simulink model "SVC"  (R2020a)
settings: Solver=VariableStepAuto  StartTime=0.0  StopTime=1  RelTol=1e-3
libraries: powerlib x7, powerlib_meascontrol x2, factslib x1
settings Model: Creator=Naeem Mohammad  LastModifiedBy=Naeem Mohammad

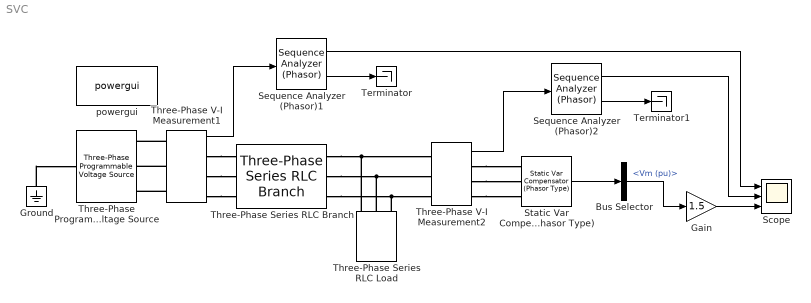
== system SVC ==
  Bus Selector : BusSelector  OutputSignals=Control.Vm (pu)
  Gain : Gain  Gain=1.5
  Ground : powerlib/Elements/Ground  LConnTagsString=a
      settings: SourceProductBaseCode=MT,PS
  Scope : Scope  NumInputPorts=3
  Sequence Analyzer (Phasor)1 : powerlib_meascontrol/Measurements/Sequence Analyzer (Phasor)  seq=Positive
      settings: SourceProductBaseCode=MT,PS
  Sequence Analyzer (Phasor)2 : powerlib_meascontrol/Measurements/Sequence Analyzer (Phasor)  seq=Positive
      settings: SourceProductBaseCode=MT,PS
  Static Var Compensator (Phasor Type) : factslib/Power-Electronics Based FACTS/Static Var Compensator (Phasor Type)  Seq1_Only=on  SystemNominal="[220  60]"  Pbase=200  Qnom="[200  -200]"  Td=4e-3  mode=Voltage regulation  Vref=1  ExternalVref=off  Xs=0.03  Kp_Ki=[0 300]  Bref=0.0
      settings: SourceProductBaseCode=PS
  Terminator : Terminator
  Terminator1 : Terminator
  Three-Phase Series RLC Branch : powerlib/Elements/Three-Phase Series RLC Branch  LConnTagsString=A|B|C  RConnTagsString=A|B|C  BranchType=RC  Resistance=220^2/300  Inductance=220^2/300/(2*pi*60)  Capacitance=(220^2/300)*(2*pi*60)  Measurements=None
      settings: SourceProductBaseCode=MT,PS
  Three-Phase Series RLC Load : powerlib/Elements/Three-Phase Series RLC Load  LConnTagsString=A|B|C  Configuration=Y (grounded)  NominalVoltage=220  Vabc=[1e3 1e3 1e3]  Vabcp=[1e3 1e3 1e3]  NominalFrequency=60  UnbalancedPower=off  ActivePower=100  InductivePower=0  CapacitivePower=10  Pabc=[10e3 9e3 11e3]  QLabc=[100 90 110]  QCabc=[100 90 110]  Pabcp=[10e3 9e3 11e3]  QLabcp=[100 90 110]  QCabcp=[100 90 110]  Measurements=None  LoadType=constant Z
      settings: SourceProductBaseCode=MT,PS
  Three-Phase V-I Measurement2 : powerlib/Measurements/Three-Phase V-I Measurement  VoltageMeasurement=phase-to-ground  SetLabelV=off  LabelV=Vabc  Vpu=on  VpuLL=off  CurrentMeasurement=no  SetLabelI=off  LabelI=Iabc  Ipu=on  Pbase=100  Vbase=220  OutputType=Complex  PhasorSimulation=on  PSBequivalent=0
  Three-Phase V-I Measurement1 : powerlib/Measurements/Three-Phase V-I Measurement  VoltageMeasurement=phase-to-ground  SetLabelV=off  LabelV=Vabc  Vpu=on  VpuLL=off  CurrentMeasurement=no  SetLabelI=off  LabelI=Iabc  Ipu=on  Pbase=100  Vbase=220  OutputType=Complex  PhasorSimulation=on  PSBequivalent=0
  Three-Phase Programmable Voltage Source : powerlib/Electrical Sources/Three-Phase Programmable Voltage Source  PositiveSequence="[220  0 60]"  VariationEntity=Amplitude  VariationType=Table of time-amplitude pairs  VariationTypeAlt=Step  VariationStep=60  VariationRate=10  VariationMagnitude=0.25  VariationFrequency=0.05  VariationTiming=[0 20]  VariationPhaseA=off  Amplitudes="[ 1  0.9  1.1  1]"  TimeValues="[ 0  0.2 0.5  0.8]"  HarmonicGeneration=off  HarmonicA=[3 0.2 -25 0]  HarmonicB=[2 0.15 35 2]  Timing="[0.05  3]"  BusType=swing  Pref=0  Qref=0  Qmin=-inf  Qmax=inf
      settings: SourceProductBaseCode=MT,PS
  powergui : powerlib/powergui  Priority=1  SimulationMode=Phasor  SampleTime=50e-6  frequency=60  Iterations=50  frequencyindice=60  Pbase=100e6  ErrMax=1e-4  UnitsV=kV  UnitsW=MW  buscounter=0  FunctionMessages=off  echomessages=off  EnableUseOfTLC=off  CurrentSourceSwitches=off  DisableSnubberDevices=off  DisableRonSwitches=off  DisableVfSwitches=off  DisplayEquations=off  AutomaticDiscreteSolvers=off  SolverType=Tustin/Backward Euler (TBE)  Interpol=off  ExternalGateDelay=off  methode=off  Ts=100  x0status=blocks  SPID=on  SwTol=0  HookPort=off  NonlinearTolerance=1e-4  nMaxIteration=100  ContinueOnMaxIteration=off  RestoreLinks=warning  ResistiveCurrentMeasurement=off  Frange=[0:2:500]  Ylog=off  Xlog=on  ShowGrid=off  save=off  variable=ZData  structure=0  ZoomFFT=off  StartTime=0.0  cycles=1  DisplayStyle=1  fundamental=60  FreqAxis=off  MaxFrequency=1000  frequencyindicesteady=1  RmsSteady=1  display=off
  wires:
  Static Var Compensator (Phasor Type)/1 -> Bus Selector/1
  Three-Phase V-I Measurement1/1 -> Sequence Analyzer (Phasor)1/1
  Sequence Analyzer (Phasor)2/1 -> Scope/2
  Sequence Analyzer (Phasor)1/1 -> Scope/1
  Three-Phase V-I Measurement2/1 -> Sequence Analyzer (Phasor)2/1
  Bus Selector/1 -> Gain/1  "<Vm (pu)>"
  Gain/1 -> Scope/3
  Sequence Analyzer (Phasor)1/2 -> Terminator/1
  Sequence Analyzer (Phasor)2/2 -> Terminator1/1
  connections:
  Three-Phase Series RLC Branch/RConn2 -- Three-Phase Series RLC Load/LConn2 -- Three-Phase V-I Measurement2/LConn2
  Three-Phase Series RLC Branch/RConn1 -- Three-Phase Series RLC Load/LConn1 -- Three-Phase V-I Measurement2/LConn1
  Three-Phase Series RLC Branch/RConn3 -- Three-Phase Series RLC Load/LConn3 -- Three-Phase V-I Measurement2/LConn3
  Ground/LConn1 -- Three-Phase Programmable Voltage Source/LConn1
  Three-Phase V-I Measurement1/LConn1 -- Three-Phase Programmable Voltage Source/RConn1
  Three-Phase V-I Measurement1/LConn2 -- Three-Phase Programmable Voltage Source/RConn2
  Three-Phase V-I Measurement1/LConn3 -- Three-Phase Programmable Voltage Source/RConn3
  Three-Phase V-I Measurement1/RConn1 -- Three-Phase Series RLC Branch/LConn1
  Three-Phase V-I Measurement1/RConn2 -- Three-Phase Series RLC Branch/LConn2
  Three-Phase V-I Measurement1/RConn3 -- Three-Phase Series RLC Branch/LConn3
  Three-Phase V-I Measurement2/RConn1 -- Static Var Compensator (Phasor Type)/LConn1
  Three-Phase V-I Measurement2/RConn2 -- Static Var Compensator (Phasor Type)/LConn2
  Three-Phase V-I Measurement2/RConn3 -- Static Var Compensator (Phasor Type)/LConn3
